simulink model "acrobot_sim_v3_PFL_non_colloc"  (R2013a)
settings: Solver=ode14x  StartTime=0.0  StopTime=10  FixedStep=0.04  RelTol=1e-3
InitFcn:
  | m1 = 1;
  | m2 = 1;
  | l1 = 1;
  | l2 = 1;
  | lc1 = l1/2;
  | lc2 = l2/2;
  | Ic1 = (lc1*lc1)/3;
  | Ic2 = (lc2*lc2)/3;
  | I1 = Ic1+m1*lc1*lc1;
  | I2 = Ic2+m2*lc2*lc2;
  | b1 = 0.4;
  | b2 = 0.4;
  | g = 9.8;
  | theta1_0 = 0;
  | theta2_0 = pi/2;
StopFcn:
  | hf = findall(0,'Name','XY Graph1'); %handle to figure window
  | ha = findall(hf,'Type','axes'); %handle to axis
  | set(ha,'XGrid','on','YGrid','on') % trun the grid on
  | set(ha,'XTick',-pi:pi/4:pi,'XTickLabel',{'-pi','-3pi/4','-pi/2','-pi/4','0','pi/4','pi/2','3pi/4','pi'});
  | 
  | hf = findall(0,'Name','XY Graph2'); %handle to figure window
  | ha = findall(hf,'Type','axes'); %handle to axis
  | set(ha,'XGrid','on','YGrid','on') % trun the grid on
  | set(ha,'XTick',-pi:pi/4:pi,'XTickLabel',{'-pi','-3pi/4','-pi/2','-pi/4','0','pi/4','pi/2','3pi/4','pi'});
libraries: mblibv1 x8, simulink x2
settings Model: Creator=nightling  LastModifiedBy=nightling
settings SimMechanicsCC: VisDuringSimulation=on

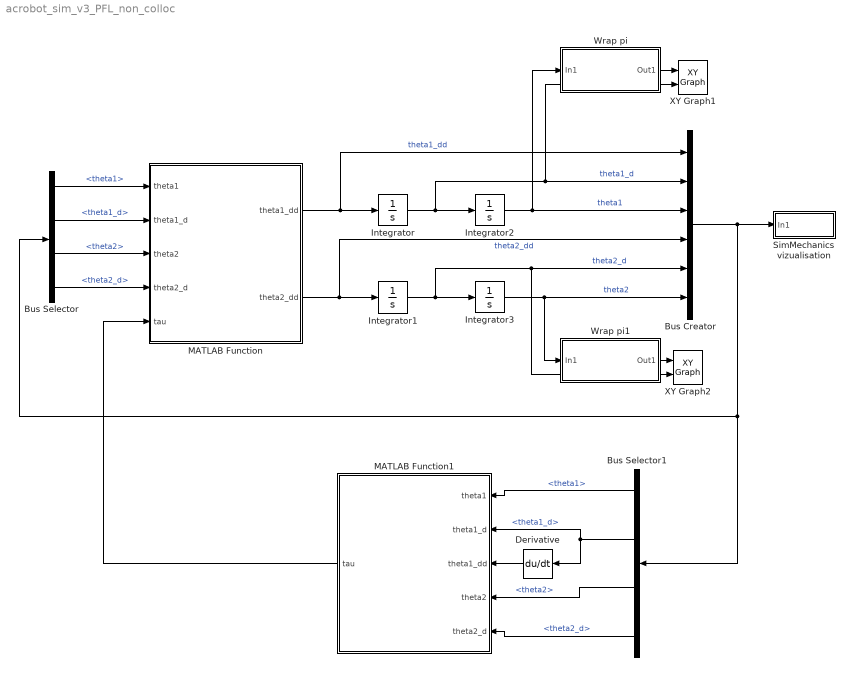
== system acrobot_sim_v3_PFL_non_colloc ==
  Bus Creator : BusCreator  Inputs=6
  Bus Selector : BusSelector  OutputSignals=theta1,theta1_d,theta2,theta2_d
  Bus Selector1 : BusSelector  OutputSignals=theta1,theta1_d,theta2,theta2_d
  Derivative : Derivative
  Integrator : Integrator  InitialCondition=[0 ]
  Integrator1 : Integrator  InitialCondition=[0 ]
  Integrator2 : Integrator  InitialCondition=theta1_0
  Integrator3 : Integrator  InitialCondition=theta2_0
  MATLAB Function : MATLAB Function  TreatAsAtomicUnit=on
  MATLAB Function1 : MATLAB Function  TreatAsAtomicUnit=on
  SimMechanics vizualisation : Subsystem
  Wrap pi : Subsystem
  Wrap pi1 : Subsystem
  XY Graph1 : simulink/Sinks/XY Graph  xmin=-pi  xmax=pi  ymin=-10  ymax=10  st=-1
  XY Graph2 : simulink/Sinks/XY Graph  xmin=-pi  xmax=pi  ymin=-10  ymax=10  st=-1
  wires:
  MATLAB Function/1(theta1_dd) -> Bus Creator/1, Integrator/1  "theta1_dd"
  MATLAB Function/2(theta2_dd) -> Integrator1/1, Bus Creator/4  "theta2_dd"
  Integrator/1 -> XY Graph1/2, Bus Creator/2, Integrator2/1  "theta1_d"
  Integrator1/1 -> Integrator3/1, XY Graph2/2, Bus Creator/5  "theta2_d"
  Integrator2/1 -> Wrap pi/1(In1), Bus Creator/3  "theta1"
  Integrator3/1 -> Wrap pi1/1(In1), Bus Creator/6  "theta2"
  Bus Creator/1 -> Bus Selector1/1, Bus Selector/1, SimMechanics vizualisation/1(In1)
  Bus Selector/1 -> MATLAB Function/1(theta1)  "<theta1>"
  Bus Selector/3 -> MATLAB Function/3(theta2)  "<theta2>"
  Bus Selector/2 -> MATLAB Function/2(theta1_d)  "<theta1_d>"
  Bus Selector/4 -> MATLAB Function/4(theta2_d)  "<theta2_d>"
  Wrap pi/1(Out1) -> XY Graph1/1
  Wrap pi1/1(Out1) -> XY Graph2/1
  MATLAB Function1/1(tau) -> MATLAB Function/5(tau)
  Bus Selector1/1 -> MATLAB Function1/1(theta1)  "<theta1>"
  Bus Selector1/2 -> Derivative/1, MATLAB Function1/2(theta1_d)  "<theta1_d>"
  Bus Selector1/3 -> MATLAB Function1/4(theta2)  "<theta2>"
  Bus Selector1/4 -> MATLAB Function1/5(theta2_d)  "<theta2_d>"
  Derivative/1 -> MATLAB Function1/3(theta1_dd)

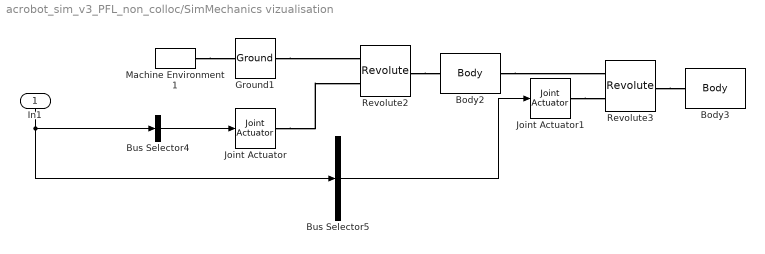
== system acrobot_sim_v3_PFL_non_colloc/SimMechanics vizualisation ==
  In1 : Inport
  Body2 : mblibv1/Bodies/Body  LConnTagsString=CS1  RConnTagsString=CS2  UpdateFromCAD=off  DialogClass=MechanicalBodyBlock  Mass=m1  MassUnits=kg  InertiaUnits=kg*m^2  Inertia=zeros(3)  Shape=Cylinder  ShapeDims=[1 1]  ShapeUnits=m  ShapeUse=false  Density=1  DensityUnits=kg/m^3  DensityUse=false  GraphicsMode=MACHINE_DEFAULT  BodyColorSelMode=COLORPALETTE  BodyColor=[0.043137 0.51765 0.78039]  AttachedToCS=CG  CG=Left$CG$[0 -l1/2 0]$CS1$CS1$m$[0 0 0]$Euler X-Y-Z$deg$WORLD$false$none  WorkingFrames=Left$CS1$[0 0 0]$Adjoining$Adjoining$m$[0 0 0]$Euler X-Y-Z$deg$WORLD$true$none#Right$CS2$[0 -l1 0]$CS1$CS1$m$[0 0 0]$Euler X-Y-Z$deg$WORLD$true$none  CGPos=[0 -l1/2 0]  CGRot=[0 0 0]  CS0Pos=[]  CS0Rot=[]  CS1Pos=[0 0 0]  CS1Rot=[0 0 0]  CS2Pos=[0 -l1 0]  CS2Rot=[0 0 0]  CS3Pos=[]  CS3Rot=[]  CS4Pos=[]  CS4Rot=[]  CS5Pos=[]  CS5Rot=[]  CS6Pos=[]  CS6Rot=[]  CS7Pos=[]  CS7Rot=[]  CS8Pos=[]  CS8Rot=[]  CS9Pos=[]  CS9Rot=[]  CS10Pos=[]  CS10Rot=[]  CS11Pos=[]  CS11Rot=[]  CS12Pos=[]  CS12Rot=[]  CS13Pos=[]  CS13Rot=[]  CS14Pos=[]  CS14Rot=[]  CS15Pos=[]  CS15Rot=[]  CS16Pos=[]  CS16Rot=[]  CS17Pos=[]  CS17Rot=[]  CS18Pos=[]  CS18Rot=[]  CS19Pos=[]  CS19Rot=[]  CS20Pos=[]  CS20Rot=[]
  Body3 : mblibv1/Bodies/Body  LConnTagsString=CS1  UpdateFromCAD=off  DialogClass=MechanicalBodyBlock  Mass=m2  MassUnits=kg  InertiaUnits=kg*m^2  Inertia=zeros(3)  Shape=Cylinder  ShapeDims=[1 1]  ShapeUnits=m  ShapeUse=false  Density=1  DensityUnits=kg/m^3  DensityUse=false  GraphicsMode=MACHINE_DEFAULT  BodyColorSelMode=COLORPALETTE  BodyColor=[0.043137 0.51765 0.78039]  AttachedToCS=CG  CG=Left$CG$[0 -l2/2 0]$CS1$CS1$m$[0 0 0]$Euler X-Y-Z$deg$WORLD$false$none  WorkingFrames=Left$CS1$[0 0 0]$Adjoining$Adjoining$m$[0 0 0]$Euler X-Y-Z$deg$WORLD$true$none#Right$CS2$[0 -l2 0]$CS1$CS1$m$[0 0 0]$Euler X-Y-Z$deg$WORLD$false$none  CGPos=[0 -l2/2 0]  CGRot=[0 0 0]  CS0Pos=[]  CS0Rot=[]  CS1Pos=[0 0 0]  CS1Rot=[0 0 0]  CS2Pos=[0 -l2 0]  CS2Rot=[0 0 0]  CS3Pos=[]  CS3Rot=[]  CS4Pos=[]  CS4Rot=[]  CS5Pos=[]  CS5Rot=[]  CS6Pos=[]  CS6Rot=[]  CS7Pos=[]  CS7Rot=[]  CS8Pos=[]  CS8Rot=[]  CS9Pos=[]  CS9Rot=[]  CS10Pos=[]  CS10Rot=[]  CS11Pos=[]  CS11Rot=[]  CS12Pos=[]  CS12Rot=[]  CS13Pos=[]  CS13Rot=[]  CS14Pos=[]  CS14Rot=[]  CS15Pos=[]  CS15Rot=[]  CS16Pos=[]  CS16Rot=[]  CS17Pos=[]  CS17Rot=[]  CS18Pos=[]  CS18Rot=[]  CS19Pos=[]  CS19Rot=[]  CS20Pos=[]  CS20Rot=[]
  Bus Selector4 : BusSelector  OutputSignals=theta1,theta1_d,theta1_dd  OutputAsBus=on
  Bus Selector5 : BusSelector  OutputSignals=theta2,theta2_d,theta2_dd  OutputAsBus=on
  Ground1 : mblibv1/Bodies/Ground  UpdateFromCAD=off  LeftPortType=env  RightPortType=workingframe  PhysicalDomain=Mechanical  DialogClass=GroundBlock  CoordPosition=[1 0 0]  CoordPositionUnits=m  StateVectorMgrId=2  MachineId=[3 0]  ShowEnvPort=on
  Joint Actuator : mblibv1/Sensors &  Actuators/Joint Actuator  UpdateFromCAD=off  PhysicalDomain=Mechanical  PortType=blob  ActuationStyle=Motion  AngleUnits=rad  ArcVelocityUnits=rad/s  ArcAccelerationUnits=rad/s^2  CoordPositionUnits=m  VelocityUnits=m/s  AccelerationUnits=m/s^2  ForceUnits=N  TorqueUnits=N*m  ActiveIO=on  Width=3  DialogClass=MechanicalActuatorBlock  Primitive=R1  ReferenceFrame=Absolute (World)
  Joint Actuator1 : mblibv1/Sensors &  Actuators/Joint Actuator  UpdateFromCAD=off  PhysicalDomain=Mechanical  PortType=blob  ActuationStyle=Motion  AngleUnits=rad  ArcVelocityUnits=rad/s  ArcAccelerationUnits=rad/s^2  CoordPositionUnits=m  VelocityUnits=m/s  AccelerationUnits=m/s^2  ForceUnits=N  TorqueUnits=N*m  ActiveIO=on  Width=3  DialogClass=MechanicalActuatorBlock  Primitive=R1  ReferenceFrame=Absolute (World)
  Machine Environment1 : mblibv1/Bodies/Machine Environment  PortType=env  PhysicalDomain=Mechanical  DialogTemplateClass=MECH.MachineEnvironment  SyncWhenCopied=off  Gravity=[0 -9.81 0]  GravityUnits=m/s^2  GravityAsSignal=off  Dimensionality=Auto-detect  AnalysisType=Forward dynamics  LinearAssemblyTolerance=1e-3  LinearAssemblyToleranceUnits=m  AngularAssemblyTolerance=1e-3  AngularAssemblyToleranceUnits=rad  ConstraintSolverType=Stabilizing  ConstraintRelTolerance=1e-4  ConstraintAbsTolerance=1e-4  UseRobustSingularityHandling=off  RedundancyAnalysisToleranceType=Automatically select tolerance  RedundancyAnalysisTolerance=1e-14  StatePerturbationType=Fixed  PerturbationSize=1e-5  VisualizeMachine=on  BodyVisualizationType=Use model default body geometries  BodyColorSelMode=Use model default  DefaultBodyColor=[1 0 0]
  Revolute2 : mblibv1/Joints/Revolute  LConnTagsString=__newl0|SA1  RConnTagsString=__newr0  UpdateFromCAD=off  NumSAPorts=1  CutJoint=off  MarkAsCut=off  Primitives=prismatic  PrimitiveProps=R1$World$[0 0 1]$revolute  DialogClass=JointBlock  R1Axis=[0 0 1]
  Revolute3 : mblibv1/Joints/Revolute  LConnTagsString=__newl0|SA1  RConnTagsString=__newr0  UpdateFromCAD=off  NumSAPorts=1  CutJoint=off  MarkAsCut=off  Primitives=prismatic  PrimitiveProps=R1$World$[0 0 1]$revolute  DialogClass=JointBlock  R1Axis=[0 0 1]
  wires:
  Bus Selector4/1 -> Joint Actuator/1
  In1/1 -> Bus Selector5/1, Bus Selector4/1
  Bus Selector5/1 -> Joint Actuator1/1
  connections:
  Revolute2/RConn1 -- Body2/LConn1
  Body2/RConn1 -- Revolute3/LConn1
  Revolute3/RConn1 -- Body3/LConn1
  Machine Environment1/RConn1 -- Ground1/LConn1
  Ground1/RConn1 -- Revolute2/LConn1
  Joint Actuator/RConn1 -- Revolute2/LConn2
  Joint Actuator1/RConn1 -- Revolute3/LConn2

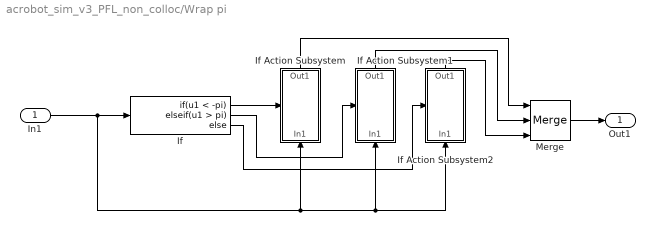
== system acrobot_sim_v3_PFL_non_colloc/Wrap pi ==
  In1 : Inport
  If : If  IfExpression=u1 < -pi  ElseIfExpressions=u1 > pi
  If Action Subsystem : Subsystem  TreatAsAtomicUnit=on
  If Action Subsystem1 : Subsystem  TreatAsAtomicUnit=on
  If Action Subsystem2 : Subsystem  TreatAsAtomicUnit=on
  Merge : Merge  Inputs=3
  Out1 : Outport
  wires:
  If/1 -> If Action Subsystem/Action
  In1/1 -> If Action Subsystem2/1(In1), If Action Subsystem1/1(In1), If Action Subsystem/1(In1), If/1
  If Action Subsystem/1(Out1) -> Merge/1
  If/2 -> If Action Subsystem1/Action
  If Action Subsystem1/1(Out1) -> Merge/2
  If Action Subsystem2/1(Out1) -> Merge/3
  If/3 -> If Action Subsystem2/Action
  Merge/1 -> Out1/1

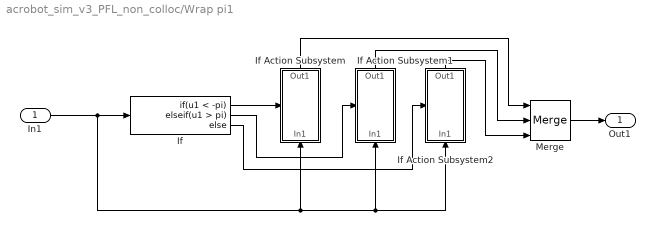
== system acrobot_sim_v3_PFL_non_colloc/Wrap pi1 ==
  In1 : Inport
  If : If  IfExpression=u1 < -pi  ElseIfExpressions=u1 > pi
  If Action Subsystem : Subsystem  TreatAsAtomicUnit=on
  If Action Subsystem1 : Subsystem  TreatAsAtomicUnit=on
  If Action Subsystem2 : Subsystem  TreatAsAtomicUnit=on
  Merge : Merge  Inputs=3
  Out1 : Outport
  wires:
  If/1 -> If Action Subsystem/Action
  In1/1 -> If Action Subsystem2/1(In1), If Action Subsystem1/1(In1), If Action Subsystem/1(In1), If/1
  If Action Subsystem/1(Out1) -> Merge/1
  If/2 -> If Action Subsystem1/Action
  If Action Subsystem1/1(Out1) -> Merge/2
  If Action Subsystem2/1(Out1) -> Merge/3
  If/3 -> If Action Subsystem2/Action
  Merge/1 -> Out1/1

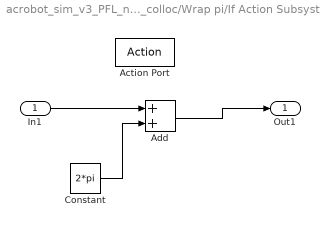
== system acrobot_sim_v3_PFL_non_colloc/Wrap pi/If Action Subsystem ==
  In1 : Inport
  Action Port : ActionPort  ActionType=then
  Add : Sum
  Constant : Constant  Value=2*pi
  Out1 : Outport
  wires:
  In1/1 -> Add/1
  Constant/1 -> Add/2
  Add/1 -> Out1/1

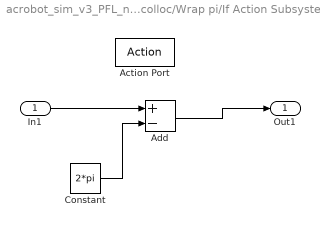
== system acrobot_sim_v3_PFL_non_colloc/Wrap pi/If Action Subsystem1 ==
  In1 : Inport
  Action Port : ActionPort  ActionType=elseif
  Add : Sum  Inputs=+-
  Constant : Constant  Value=2*pi
  Out1 : Outport
  wires:
  In1/1 -> Add/1
  Constant/1 -> Add/2
  Add/1 -> Out1/1

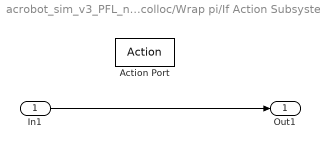
== system acrobot_sim_v3_PFL_non_colloc/Wrap pi/If Action Subsystem2 ==
  In1 : Inport
  Action Port : ActionPort  ActionType=else
  Out1 : Outport
  wires:
  In1/1 -> Out1/1

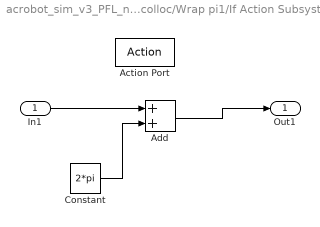
== system acrobot_sim_v3_PFL_non_colloc/Wrap pi1/If Action Subsystem ==
  In1 : Inport
  Action Port : ActionPort  ActionType=then
  Add : Sum
  Constant : Constant  Value=2*pi
  Out1 : Outport
  wires:
  In1/1 -> Add/1
  Constant/1 -> Add/2
  Add/1 -> Out1/1

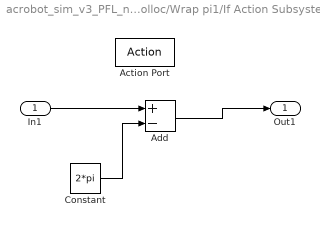
== system acrobot_sim_v3_PFL_non_colloc/Wrap pi1/If Action Subsystem1 ==
  In1 : Inport
  Action Port : ActionPort  ActionType=elseif
  Add : Sum  Inputs=+-
  Constant : Constant  Value=2*pi
  Out1 : Outport
  wires:
  In1/1 -> Add/1
  Constant/1 -> Add/2
  Add/1 -> Out1/1

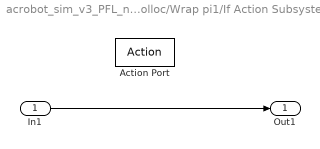
== system acrobot_sim_v3_PFL_non_colloc/Wrap pi1/If Action Subsystem2 ==
  In1 : Inport
  Action Port : ActionPort  ActionType=else
  Out1 : Outport
  wires:
  In1/1 -> Out1/1

== matlab function acrobot_sim_v3_PFL_non_colloc/MATLAB Function1 ==
  data: theta1 input; theta1_d input; theta1_dd input; theta2 input; theta2_d input; tau output
function tau  = PFL(theta1, theta1_d, theta1_dd, theta2, theta2_d)
%#codegen
    
    coder.extrinsic('PFL_non_colloc');
    tau = 0;
    
    tau = PFL_non_colloc(theta1, theta1_d, theta1_dd, theta2, theta2_d);

== matlab function acrobot_sim_v3_PFL_non_colloc/MATLAB Function ==
  data: theta1 input; theta1_dd output; theta1_d input; theta2 input; theta2_d input; theta2_dd output; tau input
function [theta1_dd, theta2_dd] = Acrobot(theta1, theta1_d, theta2, theta2_d, tau)
%#codegen
    
    coder.extrinsic('AcrobotDynamics');
    theta1_dd = 0;
    theta2_dd = 0;
    
    [theta1_dd,theta2_dd] = AcrobotDynamics(theta1, theta1_d, theta2, theta2_d, tau);
